simulink model "SHIP_UP"  (R2023a)
settings: Solver=FixedStepAuto  StartTime=0.0  StopTime=2  RelTol=1e-3
undefined symbols (not defined in the file): Cout_c, Cout_r, Cvh_c, Cvh_r, DiscIntNeverNeededParam, f, L1_l, L1_r, R_out, Uvh, Uvh_r
libraries: spsSeriesRLCBranchLib x5, spsCurrentMeasurementLib x5, spsVoltageMeasurementLib x4, simulink x2, spsDCVoltageSourceLib x1, simulink_extras x1, spsDiodeLib x1, spsMosfetLib x1, sps_lib x1
settings Model: Creator=Anton  LastModifiedBy=Александр
settings SolverCC: AlgebraicLoopSolver=TrustRegion
settings DataIOCC: ReturnWorkspaceOutputs=off
settings DebuggingCC: UnconnectedInputMsg=warning  UnconnectedOutputMsg=warning  UnconnectedLineMsg=warning  ArithmeticOperatorsInVariantConditions=warning
settings ModelReferenceCC: EnableRefExpFcnMdlSchedulingChecks=on
settings SFSimCC: SimUseLocalCustomCode=off  CustomCodeUndefinedFunction=UseInterfaceOnly
settings RTWCC: RTWUseLocalCustomCode=off
settings CodeAppCC: StateflowObjectComments=on
settings SimscapeCC: SimscapeNormalizeSystem=off

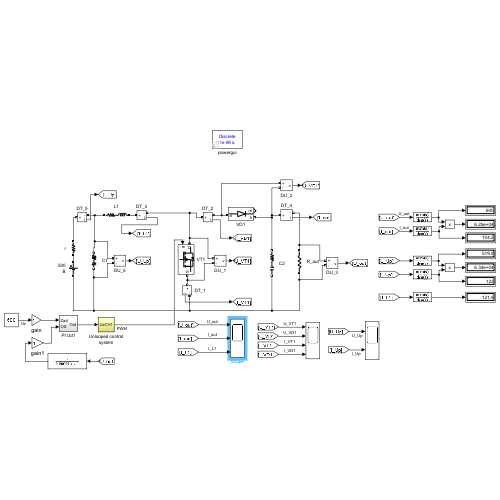
[thumbnail: Simulink's stored preview of the top-level diagram]
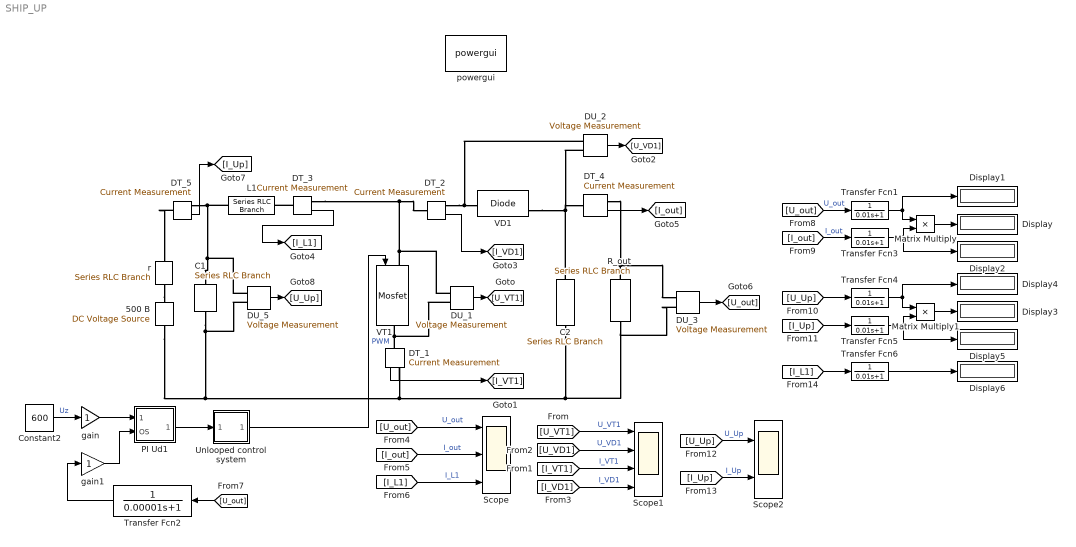
== system SHIP_UP ==
  500 В : spsDCVoltageSourceLib/DC Voltage Source  Amplitude=Uvh  Measurements=None
  C1 : spsSeriesRLCBranchLib/Series RLC Branch  LConnTagsString=__new0  RConnTagsString=__new0  BranchType=RC  Resistance=Cvh_r  Inductance=1e-3  SetiL0=off  InitialCurrent=0  Capacitance=Cvh_c  Setx0=on  InitialVoltage=Uvh  Measurements=Branch voltage
  C2 : spsSeriesRLCBranchLib/Series RLC Branch  LConnTagsString=__new0  RConnTagsString=__new0  BranchType=RC  Resistance=Cout_r  Inductance=1e-3  SetiL0=off  InitialCurrent=0  Capacitance=Cout_c  Setx0=on  InitialVoltage=Uvh  Measurements=Branch voltage
  Constant2 : Constant  Value=600
  DT_{1..5} (5 alike) : spsCurrentMeasurementLib/Current Measurement  PhasorSimulation=off  OutputType=Complex  PSBequivalent=0
  DU_{1..3,5} (4 alike) : spsVoltageMeasurementLib/Voltage Measurement  PhasorSimulation=off  OutputType=Complex  PSBequivalent=0
  Display{,1..6} (7 alike) : Display
  L1 : spsSeriesRLCBranchLib/Series RLC Branch  LConnTagsString=__new0  RConnTagsString=__new0  BranchType=RL  Resistance=L1_r  Inductance=L1_l  SetiL0=off  InitialCurrent=0  Capacitance=1e-6  Setx0=off  InitialVoltage=0  Measurements=None
  Matrix Multiply : Product
  Matrix Multiply1 : Product
  PI Ud1 : Subsystem
  R_out : spsSeriesRLCBranchLib/Series RLC Branch  LConnTagsString=__new0  RConnTagsString=__new0  BranchType=R  Resistance=R_out  Inductance=1e-3  SetiL0=off  InitialCurrent=0  Capacitance=1e-6  Setx0=off  InitialVoltage=0  Measurements=None
  Scope : Scope  NumInputPorts=3
  Scope1 : Scope  NumInputPorts=4
  Scope2 : Scope  NumInputPorts=2
  Transfer Fcn{1,3..6} (5 alike) : TransferFcn  Denominator=[0.01 1]
  Transfer Fcn2 : TransferFcn  Denominator=[0.00001 1]
  Unlooped control system : Subsystem
  VD1 : spsDiodeLib/Diode  Ron=0.001  Lon=0  Vf=1  IC=0  UseSnubber=off  Rs=inf  Cs=inf  Measurements=on
  VT1 : spsMosfetLib/Mosfet  Ron=1e-3  Lon=0  Rd=1e-3  Vfd=1  IC=0  Rs=1e5  Cs=inf  Measurements=off
  gain : Gain  SaturateOnIntegerOverflow=on  OutDataTypeStr=Inherit: Same as input  ParamDataTypeStr=Inherit: Same as input
  gain1 : Gain  SaturateOnIntegerOverflow=on  OutDataTypeStr=Inherit: Same as input  ParamDataTypeStr=Inherit: Same as input
  powergui : sps_lib/powergui  Priority=1  SimulationMode=Discrete  SampleTime=1e-6  frequency=60  Iterations=50  frequencyindice=0  Pbase=100e6  ErrMax=1e-4  UnitsV=kV  UnitsW=MW  buscounter=0  FunctionMessages=off  echomessages=off  EnableUseOfTLC=off  CurrentSourceSwitches=off  DisableSnubberDevices=off  DisableRonSwitches=off  DisableVfSwitches=off  DisplayEquations=off  AutomaticDiscreteSolvers=off  SolverType=Tustin/Backward Euler (TBE)  Interpol=off  ExternalGateDelay=off  methode=off  Ts=100  x0status=blocks  SPID=off  SwTol=0  HookPort=off  NonlinearTolerance=1e-4  nMaxIteration=100  ContinueOnMaxIteration=off  RestoreLinks=warning  ResistiveCurrentMeasurement=off  Frange=[0:2:500]  Ylog=off  Xlog=on  ShowGrid=off  save=off  variable=ZData  structure=0  ZoomFFT=off  StartTime=0.0  cycles=1  DisplayStyle=1  fundamental=60  FreqAxis=off  MaxFrequency=1000  frequencyindicesteady=1  RmsSteady=1  display=off
  r : spsSeriesRLCBranchLib/Series RLC Branch  LConnTagsString=__new0  RConnTagsString=__new0  BranchType=R  Resistance=Uvh_r  Inductance=1e-3  SetiL0=off  InitialCurrent=0  Capacitance=1e-6  Setx0=off  InitialVoltage=0  Measurements=None
  wires:
  gain/1 -> PI Ud1/1(Zad)
  gain1/1 -> PI Ud1/2(OS)
  PI Ud1/1(Out) -> Unlooped control system/1(Uz)
  Transfer Fcn2/1 -> gain1/1
  Constant2/1 -> gain/1  "Uz"
  [U_VT1] -> Scope1/1  "U_VT1"
  DU_1/1 -> [U_VT1]
  [I_VT1] -> Scope1/3  "I_VT1"
  DU_2/1 -> [U_VD1]
  [I_VD1] -> Scope1/4  "I_VD1"
  [U_VD1] -> Scope1/2  "U_VD1"
  DT_3/1 -> [I_L1]
  DT_4/1 -> [I_out]
  DU_3/1 -> [U_out]
  [U_out] -> Scope/1  "U_out"
  [I_out] -> Scope/2  "I_out"
  [U_out] -> Transfer Fcn2/1
  [I_L1] -> Scope/3  "I_L1"
  DT_2/1 -> [I_VD1]
  DT_1/1 -> [I_VT1]
  Unlooped control system/1(CH1) -> VT1/1  "PWM"
  [U_out] -> Transfer Fcn1/1  "U_out"
  [I_out] -> Transfer Fcn3/1  "I_out"
  Transfer Fcn1/1 -> Display1/1, Matrix Multiply/1
  Matrix Multiply/1 -> Display/1
  Transfer Fcn3/1 -> Display2/1, Matrix Multiply/2
  DT_5/1 -> [I_Up]
  DU_5/1 -> [U_Up]
  Transfer Fcn4/1 -> Display4/1, Matrix Multiply1/1
  Transfer Fcn5/1 -> Display5/1, Matrix Multiply1/2
  Matrix Multiply1/1 -> Display3/1
  [U_Up] -> Transfer Fcn4/1
  [I_Up] -> Transfer Fcn5/1
  [U_Up] -> Scope2/1  "U_Up"
  [I_Up] -> Scope2/2  "I_Up"
  [I_L1] -> Transfer Fcn6/1
  Transfer Fcn6/1 -> Display6/1
  connections:
  C1/RConn1 -- DU_5/LConn2 -- DT_1/RConn1 -- DU_3/LConn2 -- R_out/RConn1 -- C2/RConn1 -- 500 В/LConn1
  r/RConn1 -- 500 В/RConn1
  DT_4/RConn1 -- DU_3/LConn1 -- R_out/LConn1
  DT_3/LConn1 -- L1/RConn1
  C2/LConn1 -- DU_2/LConn2 -- DT_4/LConn1 -- VD1/RConn1
  DT_2/RConn1 -- DU_2/LConn1 -- VD1/LConn1
  L1/LConn1 -- DT_5/RConn1 -- C1/LConn1 -- DU_5/LConn1
  VT1/LConn1 -- DT_3/RConn1 -- DT_2/LConn1 -- DU_1/LConn1
  DT_1/LConn1 -- DU_1/LConn2 -- VT1/RConn1
  DT_5/LConn1 -- r/LConn1

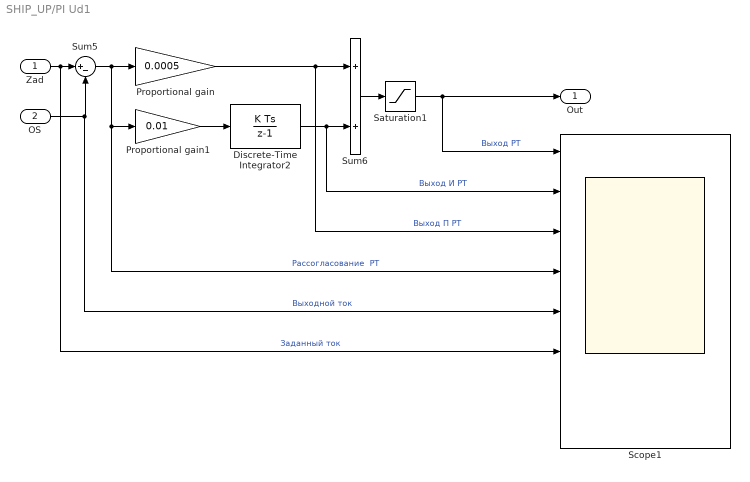
== system SHIP_UP/PI Ud1 ==
  Zad : Inport
  OS : Inport  Port=2
  Discrete-Time Integrator2 : DiscreteIntegrator  SampleTime=-1  LimitOutput=on  UpperSaturationLimit=0.9  LowerSaturationLimit=0  ICPrevOutput=DiscIntNeverNeededParam  ICPrevScaledInput=DiscIntNeverNeededParam
  Proportional gain : Gain  Gain=0.0005  SaturateOnIntegerOverflow=on  OutDataTypeStr=Inherit: Same as input  ParamDataTypeStr=Inherit: Same as input
  Proportional gain1 : Gain  Gain=0.01  SaturateOnIntegerOverflow=on  OutDataTypeStr=Inherit: Same as input  ParamDataTypeStr=Inherit: Same as input
  Saturation1 : Saturate  UpperLimit=0.9  LowerLimit=0
  Scope1 : Scope  NumInputPorts=8
  Sum5 : Sum  Inputs=|+-  InputSameDT=on  SaturateOnIntegerOverflow=on  OutDataTypeStr=Inherit: Same as first input
  Sum6 : Sum  InputSameDT=on  SaturateOnIntegerOverflow=on  OutDataTypeStr=Inherit: Same as first input
  Out : Outport  VectorParamsAs1DForOutWhenUnconnected=off
  wires:
  Proportional gain/1 -> Scope1/3, Sum6/1  "Выход П РТ"
  Discrete-Time Integrator2/1 -> Sum6/2, Scope1/2  "Выход И РТ"
  OS/1 -> Scope1/5, Sum5/2  "Выходной ток"
  Zad/1 -> Scope1/6, Sum5/1  "Заданный ток"
  Sum5/1 -> Proportional gain1/1, Scope1/4, Proportional gain/1  "Рассогласование  РТ"
  Sum6/1 -> Saturation1/1
  Saturation1/1 -> Out/1, Scope1/1  "Выход РТ"
  Proportional gain1/1 -> Discrete-Time Integrator2/1

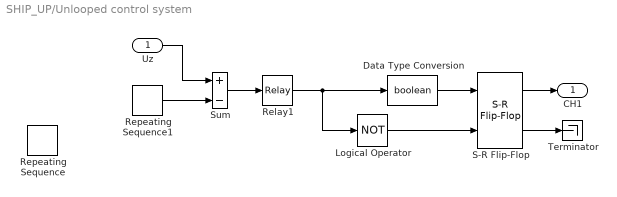
== system SHIP_UP/Unlooped control system ==
  Uz : Inport
  Data Type Conversion : DataTypeConversion  OutDataTypeStr=boolean  SaturateOnIntegerOverflow=off  RndMeth=Floor
  Logical Operator : Logic  Operator=NOT  AllPortsSameDT=off  OutDataTypeStr=boolean
  Relay1 : Relay  OnSwitchValue=0.01  OffSwitchValue=-0.01
  Repeating Sequence : simulink/Sources/Repeating Sequence  rep_seq_t=[0 0.00025]  rep_seq_y=[0 1]
  Repeating Sequence1 : simulink/Sources/Repeating Sequence  rep_seq_t="[0  (1/(2*f)) (1/f)]"  rep_seq_y=[0 1 0]
  S-R Flip-Flop : simulink_extras/Flip Flops/S-R Flip-Flop  initial_condition=0
  Sum : Sum  Inputs=+-
  Terminator : Terminator
  CH1 : Outport  VectorParamsAs1DForOutWhenUnconnected=off
  wires:
  S-R Flip-Flop/1 -> CH1/1
  Data Type Conversion/1 -> S-R Flip-Flop/1
  Logical Operator/1 -> S-R Flip-Flop/2
  Relay1/1 -> Logical Operator/1, Data Type Conversion/1
  Uz/1 -> Sum/1
  Sum/1 -> Relay1/1
  S-R Flip-Flop/2 -> Terminator/1
  Repeating Sequence1/1 -> Sum/2
